simulink model "gamler"  (Simulink 7.5)
settings: Solver=ode45  StartTime=0.0  StopTime=10.0  RelTol=1e-3
undefined symbols (not defined in the file or in its folder): magnitude
libraries: commsynccomp2 x6, powerlib_extras x4, dspxfrm3 x4, commnoisgen2 x2, commseqgen2 x2
settings Model: Creator=SISA  LastModifiedBy=SISA

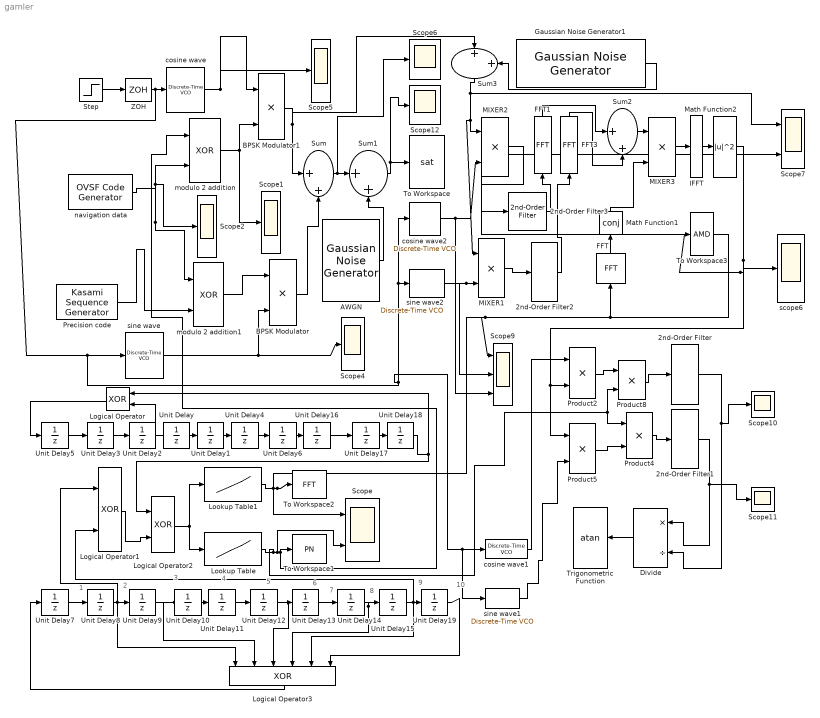
== system gamler ==
  note: 1
  note: 2
  note: 3
  note: 4
  note: 5
  note: 6
  note: 7
  note: 8
  note: 9
  note: 10
  2nd-Order Filter : powerlib_extras/Control  Blocks/2nd-Order Filter  DialogController=POWERSYS.PowerSysDialog  SystemSampleTime=-1  FilterType=Lowpass  Fo=20  Zeta=0.707  Initialize=off  Vac_Init=[1 45 60]  Vdc_Init=-0.5  PlotResponse=off  param1=[1 500 1]
  2nd-Order Filter1 : powerlib_extras/Control  Blocks/2nd-Order Filter  DialogController=POWERSYS.PowerSysDialog  SystemSampleTime=-1  FilterType=Lowpass  Fo=20  Zeta=0.707  Initialize=off  Vac_Init=[1 45 60]  Vdc_Init=-0.5  PlotResponse=off  param1=[1 500 1]
  2nd-Order Filter2 : powerlib_extras/Control  Blocks/2nd-Order Filter  DialogController=POWERSYS.PowerSysDialog  SystemSampleTime=-1  FilterType=Lowpass  Fo=15  Zeta=0.707  Initialize=off  Vac_Init=[1 45 60]  Vdc_Init=-0.5  PlotResponse=off  param1=[1 500 1]
  2nd-Order Filter3 : powerlib_extras/Control  Blocks/2nd-Order Filter  DialogController=POWERSYS.PowerSysDialog  SystemSampleTime=-1  FilterType=Lowpass  Fo=15  Zeta=0.707  Initialize=off  Vac_Init=[1 45 60]  Vdc_Init=-0.5  PlotResponse=off  param1=[1 500 1]
  AWGN : commnoisgen2/Gaussian Noise Generator  SystemSampleTime=-1  m=0  d=1  s=41  Ts=1  frameBased=off  sampPerFrame=1  orient=off  outDataType=double
  BPSK Modulator : Product  OutDataType=fixdt(1, 16)  OutScaling=2^0  RndMeth=Zero
  BPSK Modulator1 : Product  OutDataType=fixdt(1, 16)  OutScaling=2^0  RndMeth=Zero
  Divide : Product  Inputs=*/  OutDataType=fixdt(1, 16)  OutScaling=2^-10
  FFT : dspxfrm3/FFT  DialogController=dspDDGCreate  DialogControllerArgs=DataTag0  CompMethod=Table lookup  TableOpt=NEW  TableOptActive=Speed  BitRevOrder=off  InheritFFTLength=on  FFTLength=64  SkipNorm=off  firstCoeffDataTypeStr=Inherit: Same word length as input  firstCoeffLastDataTypeStr=Inherit: Same word length as input  outputMin=[]  outputMax=[]  roundingMode=Floor  overflowMode=off
  FFT1 : dspxfrm3/FFT  DialogController=dspDDGCreate  DialogControllerArgs=DataTag1  CompMethod=Table lookup  TableOpt=NEW  TableOptActive=Speed  BitRevOrder=off  InheritFFTLength=on  FFTLength=1024  SkipNorm=off  firstCoeffDataTypeStr=Inherit: Same word length as input  firstCoeffLastDataTypeStr=Inherit: Same word length as input  outputMin=[]  outputMax=[]  roundingMode=Floor  overflowMode=off
  FFT3 : dspxfrm3/FFT  DialogController=dspDDGCreate  DialogControllerArgs=DataTag2  CompMethod=Table lookup  TableOpt=NEW  TableOptActive=Speed  BitRevOrder=off  InheritFFTLength=on  FFTLength=64  SkipNorm=on  firstCoeffDataTypeStr=Inherit: Same word length as input  firstCoeffLastDataTypeStr=Inherit: Same word length as input  outputMin=[]  outputMax=[]  roundingMode=Floor  overflowMode=off
  Gaussian Noise Generator1 : commnoisgen2/Gaussian Noise Generator  SystemSampleTime=-1  m=0  d=1  s=41  Ts=1  frameBased=off  sampPerFrame=1  orient=off  outDataType=double
  IFFT : dspxfrm3/IFFT  DialogController=dspDDGCreate  DialogControllerArgs=DataTag3  CompMethod=Table lookup  TableOpt=NEW  TableOptActive=Speed  BitRevOrder=on  cs_in=off  SkipNorm=off  InheritFFTLength=on  FFTLength=1024  mode=Complex  outSamplingMode=Sample based  firstCoeffDataTypeStr=Inherit: Same word length as input  firstCoeffLastDataTypeStr=Inherit: Same word length as input  outputMin=[]  outputMax=[]  roundingMode=Floor  overflowMode=off
  Logical Operator : Logic  Operator=XOR  AllPortsSameDT=off  OutDataTypeMode=boolean  LogicDataType=fixdt(0, 8)  OutDataTypeStr=boolean
  Logical Operator1 : Logic  Operator=XOR  AllPortsSameDT=off  OutDataTypeMode=boolean  LogicDataType=fixdt(0, 8)  OutDataTypeStr=boolean
  Logical Operator2 : Logic  Operator=XOR  AllPortsSameDT=off  OutDataTypeMode=boolean  LogicDataType=fixdt(0, 8)  OutDataTypeStr=boolean
  Logical Operator3 : Logic  Operator=XOR  Inputs=6  AllPortsSameDT=off  OutDataTypeMode=boolean  LogicDataType=fixdt(0, 8)  OutDataTypeStr=boolean
  Lookup Table : Lookup  InputValues=[0,1]  Table=[0,1]  LookUpMeth=Use Input Above  OutDataType=fixdt(1, 16)  OutScaling=2^0
  Lookup Table1 : Lookup  InputValues=[0,1]  Table=[0,1]  LookUpMeth=Use Input Nearest  OutDataTypeMode=double  OutDataType=fixdt(1, 16)  OutScaling=2^0  OutDataTypeStr=double  RndMeth=Zero
  MIXER1 : Product  OutDataType=fixdt(1, 16)  OutScaling=2^0  RndMeth=Zero
  MIXER2 : Product  OutDataType=fixdt(1, 16)  OutScaling=2^0  RndMeth=Zero
  MIXER3 : Product  OutDataType=fixdt(1, 16)  OutScaling=2^0  RndMeth=Zero
  Math Function1 : Math  Operator=conj  OutputSignalType=complex  OutDataType=fixdt(1, 16)  OutScaling=2^0  SaturateOnIntegerOverflow=on
  Math Function2 : Math  Operator=magnitude^2  OutDataType=fixdt(1, 16)  OutScaling=2^0  SaturateOnIntegerOverflow=on
  Precision code : commseqgen2/Kasami Sequence Generator  genPoly=[1 0 1 0 0 1 1]  iniState=[0 0 0 0 0 1]  codeIdx=0  shift=0  ts=1  frameBased=off  sampPerFrame=1  reset=off  outDataType=double
  Product{2,4..5,8} (4 alike) : Product  OutDataType=fixdt(1, 16)  OutScaling=2^0  RndMeth=Zero
  Scope : Scope  NumInputPorts=2
      settings: TimeRange=10  YMin=-5~-5  YMax=5~5  SaveName=ScopeData6  SampleInput=on
  Scope{1..2,4..6,10..12} (8 alike) : Scope
      Scope10 settings: SaveName=ScopeData10
      Scope11 settings: SaveName=ScopeData11
      Scope12 settings: SaveName=ScopeData12
      Scope4 settings: SaveName=ScopeData3
      Scope5 settings: SaveName=ScopeData4
      Scope6 settings: SaveName=ScopeData5
  Scope7 : Scope  NumInputPorts=2
      settings: YMin=-5~-5  YMax=5~5  SaveName=ScopeData7
  Scope9 : Scope  NumInputPorts=3
      settings: YMin=-2~-5~-5  YMax=2~5~5  SaveName=ScopeData9
  Step : Step  After=3  SampleTime=0
  Sum{,1..3} (4 alike) : Sum  Inputs=|++  OutDataType=fixdt(1, 16)  OutScaling=2^0
  To Workspace : ToWorkspace  VariableName=sat  SampleTime=-1  SaveFormat=Array
      settings: MaxDataPoints=1023000
  To Workspace1 : ToWorkspace  VariableName=PN  SampleTime=-1  SaveFormat=Array
      settings: MaxDataPoints=1023000
  To Workspace2 : ToWorkspace  VariableName=FFT  SampleTime=-1  SaveFormat=Array
      settings: MaxDataPoints=1023000
  To Workspace3 : ToWorkspace  VariableName=AMD  SampleTime=-1  SaveFormat=Array
      settings: MaxDataPoints=1023000
  Trigonometric Function : Trigonometry  Operator=atan
  Unit Delay{,1..19} (20 alike) : UnitDelay  X0=1  SampleTime=-1
  ZOH : ZeroOrderHold
  cosine wave : commsynccomp2/Discrete-Time VCO  SystemSampleTime=-1  Ac=3  Fc=7000000  Kc=1  Ph=0.02  ts=0.01
  cosine wave1 : commsynccomp2/Discrete-Time VCO  SystemSampleTime=-1  Ac=3  Fc=7000000  Kc=1  Ph=0  ts=0.01
  cosine wave2 : commsynccomp2/Discrete-Time VCO  SystemSampleTime=-1  Ac=3  Fc=7000000  Kc=1  Ph=0  ts=0.01
  modulo 2 addition : Logic  Operator=XOR  IconShape=distinctive  AllPortsSameDT=off  OutDataTypeMode=boolean  LogicDataType=fixdt(0, 8)  OutDataTypeStr=boolean
  modulo 2 addition1 : Logic  Operator=XOR  IconShape=distinctive  AllPortsSameDT=off  OutDataTypeMode=boolean  LogicDataType=fixdt(0, 8)  OutDataTypeStr=boolean
  navigation data : commseqgen2/OVSF Code Generator  SystemSampleTime=-1  spreadFact=64  index=61  ts=0.1  frameBased=off  sampPerFrame=1  outDataType=double
  scope6 : Scope
      settings: TimeRange=10  YMin=0  YMax=100  SaveName=ScopeData8
  sine wave : commsynccomp2/Discrete-Time VCO  SystemSampleTime=-1  Ac=3  Fc=7000000  Kc=1  Ph=-pi/2 + 0.02  ts=0.01
  sine wave1 : commsynccomp2/Discrete-Time VCO  SystemSampleTime=-1  Ac=3  Fc=7000000  Kc=1  Ph=-pi/2  ts=0.01
  sine wave2 : commsynccomp2/Discrete-Time VCO  SystemSampleTime=-1  Ac=3  Fc=7000000  Kc=1  Ph=-pi/2  ts=0.01
  wires:
  BPSK Modulator1/1 -> Sum/1, Sum3/1
  modulo 2 addition/1 -> BPSK Modulator1/2, Scope1/1
  Step/1 -> ZOH/1
  ZOH/1 -> cosine wave/1, sine wave/1, sine wave2/1, cosine wave2/1, cosine wave1/1, sine wave1/1
  cosine wave/1 -> BPSK Modulator1/1, Scope5/1
  navigation data/1 -> modulo 2 addition1/1, modulo 2 addition/2, Scope2/1
  modulo 2 addition1/1 -> BPSK Modulator/1
  sine wave/1 -> BPSK Modulator/2, Scope4/1
  BPSK Modulator/1 -> Sum/2
  Sum/1 -> Sum1/1, Scope6/1
  AWGN/1 -> Sum1/2
  Sum1/1 -> Scope12/1, To Workspace/1
  FFT1/1 -> Sum2/1
  FFT3/1 -> Sum2/2
  Math Function1/1 -> MIXER3/2
  FFT/1 -> Math Function1/1
  Math Function2/1 -> To Workspace3/1, Product2/2, Product5/1, scope6/1
  Sum2/1 -> MIXER3/1
  IFFT/1 -> Math Function2/1
  MIXER3/1 -> IFFT/1
  Unit Delay3/1 -> Unit Delay2/1
  Unit Delay2/1 -> Unit Delay/1, Logical Operator/2
  Unit Delay/1 -> Unit Delay1/1
  Unit Delay1/1 -> Unit Delay4/1
  Unit Delay5/1 -> Unit Delay3/1
  Unit Delay4/1 -> Unit Delay6/1
  Unit Delay6/1 -> Unit Delay16/1
  Unit Delay16/1 -> Unit Delay17/1
  Unit Delay17/1 -> Unit Delay18/1
  Unit Delay7/1 -> Unit Delay8/1
  Unit Delay9/1 -> Logical Operator3/2, Unit Delay10/1
  Unit Delay10/1 -> Unit Delay11/1
  Unit Delay11/1 -> Unit Delay12/1
  Unit Delay12/1 -> Logical Operator3/3, Unit Delay13/1
  Unit Delay13/1 -> Unit Delay14/1
  Unit Delay14/1 -> Logical Operator3/4, Unit Delay15/1
  Logical Operator/1 -> Unit Delay5/1
  Logical Operator2/1 -> Lookup Table/1, Lookup Table1/1
  Unit Delay18/1 -> Logical Operator2/1, Logical Operator/1
  Logical Operator1/1 -> Logical Operator2/2
  Logical Operator3/1 -> Unit Delay7/1
  Unit Delay19/1 -> Logical Operator3/6
  Unit Delay8/1 -> Logical Operator3/1, Unit Delay9/1, Logical Operator1/1
  Lookup Table/1 -> Scope/2, To Workspace1/1, modulo 2 addition/1, Product8/2, Product4/1
  Lookup Table1/1 -> To Workspace2/1, Scope/1, Scope9/1, Scope7/2, FFT/1
  Gaussian Noise Generator1/1 -> Sum3/2
  Sum3/1 -> Scope7/1, MIXER2/1, MIXER1/1
  Precision code/1 -> modulo 2 addition1/2
  Unit Delay15/1 -> Unit Delay19/1, Logical Operator3/5, Logical Operator1/2
  MIXER1/1 -> 2nd-Order Filter2/1
  2nd-Order Filter2/1 -> FFT3/1
  MIXER2/1 -> 2nd-Order Filter3/1
  2nd-Order Filter3/1 -> FFT1/1
  2nd-Order Filter/1 -> Divide/2, Scope10/1
  2nd-Order Filter1/1 -> Scope11/1, Divide/1
  Product4/1 -> 2nd-Order Filter1/1
  Product8/1 -> 2nd-Order Filter/1
  Divide/1 -> Trigonometric Function/1
  Product5/1 -> Product4/2
  Product2/1 -> Product8/1
  sine wave1/1 -> Product5/2
  cosine wave2/1 -> MIXER2/2, Scope9/3
  sine wave2/1 -> MIXER1/2, Scope9/2
  cosine wave1/1 -> Product2/1
